simulink model "desing"  (R2024a)
settings: Solver=VariableStepAuto  StartTime=0.0  StopTime=10.0  RelTol=1e-3
libraries: spsThyristorLib x6, spsACVoltageSourceLib x3, spsThreePhaseVIMeasurementLib x3, spsGroundLib x2, spsThreePhaseBreakerLib x2, spsAlphaBetaZerotodq0Lib x1, slpidlib x1, spsabctoAlphaBetaZeroLib x1, spsThreePhaseParallelRLCBranchLib x1, sps_lib x1
settings Model: Creator=gshma  LastModifiedBy=gshma

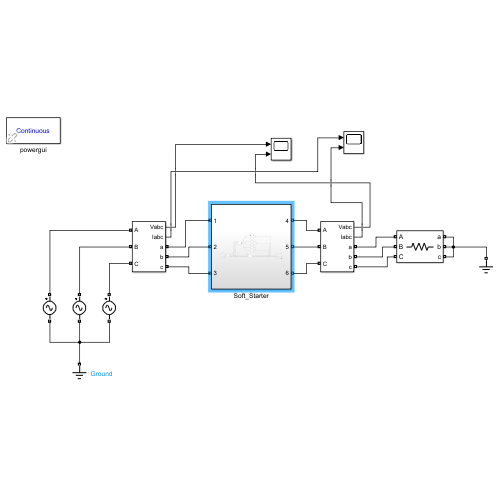
[thumbnail: Simulink's stored preview of the top-level diagram]
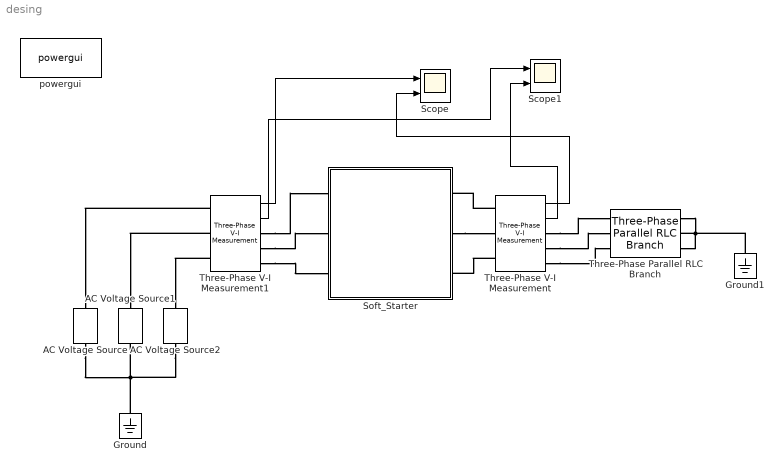
== system desing ==
  AC Voltage Source : spsACVoltageSourceLib/AC Voltage Source  Amplitude=400  Phase=0  Frequency=50  SampleTime=0  Measurements=None  BusType=swing  Pref=10e3  Qref=0  Qmin=-inf  Qmax=+inf
  AC Voltage Source1 : spsACVoltageSourceLib/AC Voltage Source  Amplitude=400  Phase=120  Frequency=50  SampleTime=0  Measurements=None  BusType=swing  Pref=10e3  Qref=0  Qmin=-inf  Qmax=+inf
  AC Voltage Source2 : spsACVoltageSourceLib/AC Voltage Source  Amplitude=400  Phase=240  Frequency=50  SampleTime=0  Measurements=None  BusType=swing  Pref=10e3  Qref=0  Qmin=-inf  Qmax=+inf
  Ground : spsGroundLib/Ground  LConnTagsString=a
  Ground1 : spsGroundLib/Ground  LConnTagsString=a
  Scope : Scope  NumInputPorts=2
  Scope1 : Scope  NumInputPorts=2
  Soft_Starter : Subsystem
  Three-Phase Parallel RLC Branch : spsThreePhaseParallelRLCBranchLib/Three-Phase Parallel RLC Branch  LConnTagsString=A|B|C  RConnTagsString=A|B|C  BranchType=R  Resistance=10  Inductance=1e-3  Capacitance=1e-6  Measurements=None
  Three-Phase V-I Measurement : spsThreePhaseVIMeasurementLib/Three-Phase V-I Measurement  VoltageMeasurement=phase-to-phase  SetLabelV=off  LabelV=Vabc  Vpu=off  VpuLL=off  CurrentMeasurement=yes  SetLabelI=off  LabelI=Iabc  Ipu=off  Pbase=100e6  Vbase=500e3  OutputType=Complex  PhasorSimulation=off  PSBequivalent=0
  Three-Phase V-I Measurement1 : spsThreePhaseVIMeasurementLib/Three-Phase V-I Measurement  VoltageMeasurement=phase-to-phase  SetLabelV=off  LabelV=Vabc  Vpu=off  VpuLL=off  CurrentMeasurement=yes  SetLabelI=off  LabelI=Iabc  Ipu=off  Pbase=100e6  Vbase=500e3  OutputType=Complex  PhasorSimulation=off  PSBequivalent=0
  powergui : sps_lib/powergui  Priority=1  SimulationMode=Continuous  SampleTime=50e-6  frequency=60  Iterations=50  frequencyindice=50  Pbase=100e6  ErrMax=1e-4  UnitsV=kV  UnitsW=MW  buscounter=0  FunctionMessages=off  echomessages=off  EnableUseOfTLC=off  CurrentSourceSwitches=off  DisableSnubberDevices=off  DisableRonSwitches=off  DisableVfSwitches=off  DisplayEquations=off  AutomaticDiscreteSolvers=off  SolverType=Tustin/Backward Euler (TBE)  Interpol=off  ExternalGateDelay=off  methode=off  Ts=100  x0status=blocks  SPID=on  SwTol=0  HookPort=off  NonlinearTolerance=1e-4  nMaxIteration=100  ContinueOnMaxIteration=off  RestoreLinks=warning  ResistiveCurrentMeasurement=off  Frange=[0:2:500]  Ylog=off  Xlog=on  ShowGrid=off  save=off  variable=ZData  structure=0  ZoomFFT=off  StartTime=0.0  cycles=1  DisplayStyle=1  fundamental=60  FreqAxis=off  MaxFrequency=1000  frequencyindicesteady=1  RmsSteady=1  display=off
  wires:
  Three-Phase V-I Measurement/1 -> Scope/2
  Three-Phase V-I Measurement1/1 -> Scope/1
  Three-Phase V-I Measurement1/2 -> Scope1/1
  Three-Phase V-I Measurement/2 -> Scope1/2
  connections:
  AC Voltage Source/LConn1 -- Ground/LConn1 -- AC Voltage Source2/LConn1 -- AC Voltage Source1/LConn1
  Three-Phase Parallel RLC Branch/RConn1 -- Ground1/LConn1 -- Three-Phase Parallel RLC Branch/RConn3 -- Three-Phase Parallel RLC Branch/RConn2
  Soft_Starter/RConn2 -- Three-Phase V-I Measurement/LConn2
  Three-Phase V-I Measurement/LConn1 -- Soft_Starter/RConn1
  Three-Phase V-I Measurement/LConn3 -- Soft_Starter/RConn3
  Three-Phase V-I Measurement/RConn1 -- Three-Phase Parallel RLC Branch/LConn1
  Three-Phase V-I Measurement/RConn2 -- Three-Phase Parallel RLC Branch/LConn2
  Three-Phase V-I Measurement/RConn3 -- Three-Phase Parallel RLC Branch/LConn3
  Three-Phase V-I Measurement1/RConn2 -- Soft_Starter/LConn2
  Three-Phase V-I Measurement1/RConn1 -- Soft_Starter/LConn1
  Three-Phase V-I Measurement1/RConn3 -- Soft_Starter/LConn3
  Three-Phase V-I Measurement1/LConn1 -- AC Voltage Source/RConn1
  Three-Phase V-I Measurement1/LConn2 -- AC Voltage Source1/RConn1
  Three-Phase V-I Measurement1/LConn3 -- AC Voltage Source2/RConn1

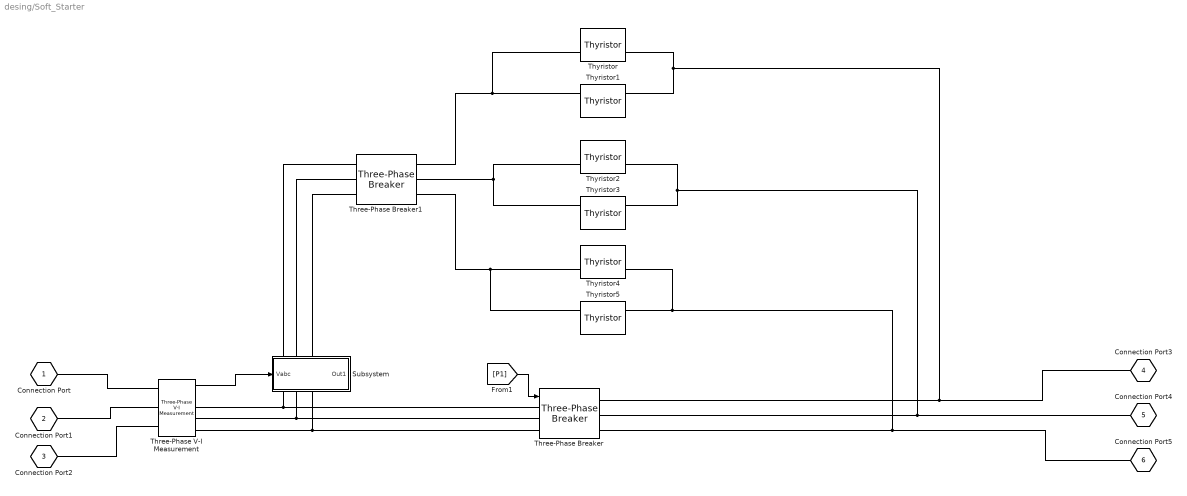
== system desing/Soft_Starter ==
  Subsystem : Subsystem
  Three-Phase V-I Measurement : spsThreePhaseVIMeasurementLib/Three-Phase V-I Measurement  VoltageMeasurement=phase-to-phase  SetLabelV=off  LabelV=Vabc  Vpu=off  VpuLL=off  CurrentMeasurement=yes  SetLabelI=off  LabelI=Iabc  Ipu=off  Pbase=100e6  Vbase=500e3  OutputType=Complex  PhasorSimulation=off  PSBequivalent=0
  Three-Phase Breaker : spsThreePhaseBreakerLib/Three-Phase Breaker  InitialState=open  SwitchA=on  SwitchB=on  SwitchC=on  SwitchTimes="[1/60  5/60]"  External=on  BreakerResistance=0.01  SnubberResistance=1e6  SnubberCapacitance=inf  Measurements=None
  Three-Phase Breaker1 : spsThreePhaseBreakerLib/Three-Phase Breaker  InitialState=closed  SwitchA=on  SwitchB=on  SwitchC=on  SwitchTimes="[1/60  5/60]"  External=off  BreakerResistance=0.01  SnubberResistance=1e6  SnubberCapacitance=inf  Measurements=None
  Thyristor{,1..5} (6 alike) : spsThyristorLib/Thyristor  Ron=0.001  Lon=0  Vf=0.8  IC=0  Rs=500  Cs=250e-9  Measurements=on
  Connection Port : PMIOPort  Tag=simrfV2util1/Connection Port  Side=Left
  Connection Port1 : PMIOPort  Tag=simrfV2util1/Connection Port  Port=2  Side=Left
  Connection Port2 : PMIOPort  Tag=simrfV2util1/Connection Port  Port=3  Side=Left
  Connection Port3 : PMIOPort  Tag=simrfV2util1/Connection Port  Port=4  Side=Right
  Connection Port4 : PMIOPort  Tag=simrfV2util1/Connection Port  Port=5  Side=Right
  Connection Port5 : PMIOPort  Tag=simrfV2util1/Connection Port  Port=6  Side=Right
  wires:
  [P1] -> Three-Phase Breaker/1
  Three-Phase V-I Measurement/1 -> Subsystem/1(Vabc)
  connections:
  Three-Phase Breaker1/LConn2 -- Three-Phase Breaker/LConn2 -- Three-Phase V-I Measurement/RConn2
  Three-Phase Breaker1/LConn1 -- Three-Phase V-I Measurement/RConn1 -- Three-Phase Breaker/LConn1
  Thyristor4/RConn1 -- Three-Phase Breaker/RConn3 -- Connection Port5/RConn1 -- Thyristor5/LConn1
  Three-Phase Breaker1/LConn3 -- Three-Phase V-I Measurement/RConn3 -- Three-Phase Breaker/LConn3
  Thyristor1/LConn1 -- Connection Port3/RConn1 -- Three-Phase Breaker/RConn1 -- Thyristor/RConn1
  Thyristor2/RConn1 -- Three-Phase Breaker/RConn2 -- Connection Port4/RConn1 -- Thyristor3/LConn1
  Thyristor1/RConn1 -- Three-Phase Breaker1/RConn1 -- Thyristor/LConn1
  Thyristor5/RConn1 -- Three-Phase Breaker1/RConn3 -- Thyristor4/LConn1
  Thyristor2/LConn1 -- Thyristor3/RConn1 -- Three-Phase Breaker1/RConn2
  Connection Port/RConn1 -- Three-Phase V-I Measurement/LConn1
  Connection Port1/RConn1 -- Three-Phase V-I Measurement/LConn2
  Connection Port2/RConn1 -- Three-Phase V-I Measurement/LConn3

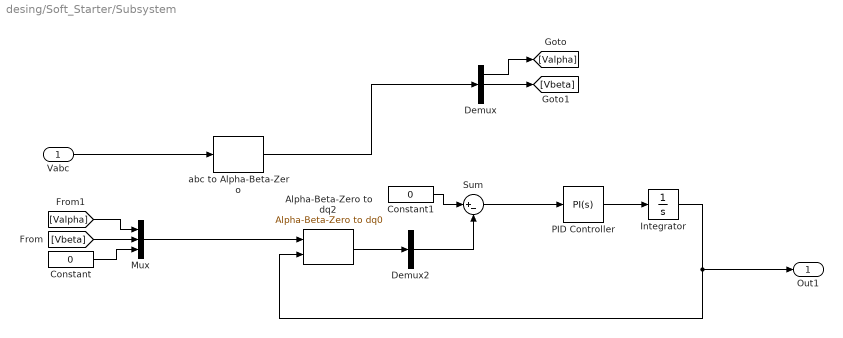
== system desing/Soft_Starter/Subsystem ==
  Vabc : Inport
  Alpha-Beta-Zero to dq2 : spsAlphaBetaZerotodq0Lib/Alpha-Beta-Zero to dq0  Alignment=90 degrees behind phase A axis
  Constant : Constant  Value=0  SampleTime=0.000001
  Constant1 : Constant  Value=0  SampleTime=0.000001
  Demux : Demux  Outputs=3
  Demux2 : Demux  Outputs=3
  Integrator : Integrator
  Mux : Mux  Inputs=3
  PID Controller : slpidlib/PID Controller  Controller=PI  Form=Parallel  TimeDomain=Continuous-time  UseExternalTs=off  SampleTime=-1  IntegratorMethod=Forward Euler  FilterMethod=Forward Euler  ControllerParametersSource=internal  P=10  I=50000  UseKiTs=off  D=0  UseExternalDerivativeSource=off  N=100  UseFilter=on  TunerSelectOption=Transfer Function Based (PID Tuner App)  InitialConditionSource=internal  InitialConditionForIntegrator=0  InitialConditionForFilter=0  DifferentiatorICPrevScaledInput=0  ExternalReset=none  TrackingMode=off  Kt=1  LimitOutput=off  SatLimitsSource=internal  UpperSaturationLimit=inf  LowerSaturationLimit=-inf  LinearizeAsGain=on  AntiWindupMode=none  Kb=1  LimitIntegrator=off  UpperIntegratorSaturationLimit=inf  LowerIntegratorSaturationLimit=-inf  POutMin=[]  POutMax=[]  IOutMin=[]  IOutMax=[]  DOutMin=[]  DOutMax=[]  NOutMin=[]  NOutMax=[]  SumOutMin=[]  SumOutMax=[]  SaturationOutMin=[]  SaturationOutMax=[]  PParamMin=[]  PParamMax=[]  IParamMin=[]  IParamMax=[]  DParamMin=[]  DParamMax=[]  NParamMin=[]  NParamMax=[]  KbParamMin=[]  KbParamMax=[]  KtParamMin=[]  KtParamMax=[]  KbOutMin=[]  KbOutMax=[]  KtOutMin=[]  KtOutMax=[]  IntegratorOutMin=[]  IntegratorOutMax=[]  FilterOutMin=[]  FilterOutMax=[]  SumI1OutMin=[]  SumI1OutMax=[]  SumI2OutMin=[]  SumI2OutMax=[]  SumI3OutMin=[]  SumI3OutMax=[]  SumI4OutMin=[]  SumI4OutMax=[]  SumDOutMin=[]  SumDOutMax=[]  DifferentiatorOutMin=[]  DifferentiatorOutMax=[]  FilterDiffOutCoefMin=[]  FilterDiffOutCoefMax=[]  ReciprocalOutMin=[]  ReciprocalOutMax=[]  SumDenOutMin=[]  SumDenOutMax=[]  SumNumOutMin=[]  SumNumOutMax=[]  DivideOutMin=[]  DivideOutMax=[]  UdiffTsProdOutMin=[]  UdiffTsProdOutMax=[]  NTsProdOutMin=[]  NTsProdOutMax=[]  UintegralTsProdOutMin=[]  UintegralTsProdOutMax=[]  UngainTsProdOutMin=[]  UngainTsProdOutMax=[]  ClampingZeroOutDataTypeStr=Inherit: Inherit via back propagation  ClampingZeroOutMin=[]  ClampingZeroOutMax=[]  FilterDenConstantOutDataTypeStr=Inherit: Inherit via back propagation  FilterDenConstantOutMin=[]  FilterDenConstantOutMax=[]  PCopyOutDataTypeStr=Inherit: Inherit via back propagation  PCopyOutMin=[]  PCopyOutMax=[]  NCopyOutDataTypeStr=Inherit: Inherit via back propagation  NCopyOutMin=[]  NCopyOutMax=[]  IntegratorContinuousStateAttributes=''  IntegratorStateMustResolveToSignalObject=off  IntegratorRTWStateStorageClass=Auto  FilterContinuousStateAttributes=''  FilterStateMustResolveToSignalObject=off  FilterRTWStateStorageClass=Auto  ParallelPVariant=InternalParameters  IdealPVariant=Disabled  IVariant=InternalParameters  DVariant=Disabled  IntegratorVariant=Continuous  SatVariant=Disabled  AWVariant=Passthrough  PCopyVariant=Disabled  TRVariant=Disabled  FdbkBlocksVariant=Forward  IdealPFdbkVariant=Disabled  SatFdbkVariant=Disabled  DerivativeFilterVariant=Disabled  NVariant=Disabled  NCopyVariant=Disabled_SignalSpec  FilterICVariant=Disabled  IntegratorICVariant=InternalICs  ExternalResetVariant=Disabled  TRSumVariant=Passthrough  SumFdbkVariant=Disabled  SumVariant=Sum_PI  TsampFilterVariant=InternalTs  TsampNgainVariant=Passthrough  TsampIntegralVariant=Disabled_SignalSpec  ExternalSaturationOutDataTypeStr=Inherit: Same as second input  DerivativeSourceVariant=Disabled
  Sum : Sum  Inputs=|+-
  abc to Alpha-Beta-Zero : spsabctoAlphaBetaZeroLib/abc to Alpha-Beta-Zero
  Out1 : Outport
  wires:
  Vabc/1 -> abc to Alpha-Beta-Zero/1
  abc to Alpha-Beta-Zero/1 -> Demux/1
  Demux/1 -> [Valpha]
  Demux/2 -> [Vbeta]
  [Vbeta] -> Mux/2
  Constant/1 -> Mux/3
  Mux/1 -> Alpha-Beta-Zero to dq2/1
  [Valpha] -> Mux/1
  Demux2/2 -> Sum/2
  Alpha-Beta-Zero to dq2/1 -> Demux2/1
  Constant1/1 -> Sum/1
  Sum/1 -> PID Controller/1
  PID Controller/1 -> Integrator/1
  Integrator/1 -> Alpha-Beta-Zero to dq2/2, Out1/1
